simulink model "CusakisME4901arcs2"  (R2013a)
settings: Solver=ode4  StartTime=0.0  StopTime=inf  FixedStep=0.01  RelTol=1e-3
InitFcn:
  | start_EEVSCube2
  | 
  | %links masses
  | 
  | m=20;%Kg
  | 
  | l=1;%meter
  | 
  | w=0.08;
  | 
  | I=(1/12)*m*(l^2); %moment of inertia
  | 
  | %estimation error
  | 
  | mn=20+m*0.05;
  | In=I+I*0.1;
  | 
  | %controls
  | 
  | a=0.7; %singularity positive gain
  | 
  | %Chaser
  | mb=100;%kg
  | lc=2;%meters
  | lb=lc/2;%meter distance 1joint to CM
  | Ib=(1/12)*mb*(lc^2+lc^2);
  | 
  | %Target
  | 
  | mt=750;%kg target mass
  | lt=1;%meter  side lenght
  | It=(1/6)*(lt^2)*mt;
  | 
  | %Target Initial Conitions
  | 
  | x_t=2;
  | y_t=2;
  | theta_t=0.7853;
  | 
  | Init_t=[x_t;y_t;theta_t;0;0;0];
  | Iinv=pinv(eye(3)*It);
StopFcn:
  | figure(1)
  | subplot(2,1,1)
  | hold on
  | plot(time,kinetic,'g')
  | grid on
  | title('Kinetic Energy vs Time')
  | xlabel('Time')
  | ylabel('Kinetic Energy')
  | hold off
  | 
  | subplot(2,1,2)
  | hold on
  | plot(time,power,'g')
  | grid on
  | title('Power Consumption vs Time')
  | xlabel('Time')
  | ylabel('Power')
  | hold off
  | 
  | chasermapping=[-1,1;-1,-1;1,-1;1,1;-1,1];
  | targetmapping=[1.293,2;2,2.707;2.707,2;2,1.293;1.293,2];
  | 
  | figure(3)
  | hold on
  | plot(EEstate(:,1),EEstate(:,2),'g')
  | plot(targetmapping(:,1),targetmapping(:,2),'r')
  | plot(chasermapping(:,1),chasermapping(:,2),'b')
  | grid on
  | title('End Effector Path')
  | xlabel('X Axis (m)')
  | ylabel('Y Axis (m)')
  | hold off
  | 
  | 
  | figure(4)
  | subplot(2,1,1)
  | hold on
  | plot(time,qqd(:,1),'g')
  | plot(time,qqd(:,2),'r')
  | plot(time,qqd(:,3),'b')
  | grid on
  | title('Theta vs Time')
  | xlabel('Time (sec)')
  | ylabel('Theta (rad)')
  | legend( 'Theta1 ' , ' Theta2 ' , ' Theta3')
  | hold off
  | 
  | subplot(2,1,2)
  | hold on
  | plot(time,qqd(:,4),'g')
  | plot(time,qqd(:,5),'r')
  | plot(time,qqd(:,6),'b')
  | grid on
  | legend( 'Omega1 ' , ' Omega2 ', ' Omega3 ' )
  | title('Omega vs Time')
  | xlabel('Time (sec)')
  | ylabel('Omega (rad/s)')
values from neighbouring files (symbols this model uses):
  D = sqrt((Xf(1)-Xi(1))^2+(Xf(2)-Xi(2))^2)    [Arcpaths.m]
undefined symbols (not defined in the file or in its folder): mesh_A, mesh_B, serial
libraries: instrumentlib x5, simulink x3, vrlib x2, dspinverses x1, aerolibanimutils x1
(part 4 of 4)

== matlab function CusakisME4901arcs2/Hardware Interface Comuincation/rad to Arm/MATLAB Function3 ==
  data: u input; y output
function y = fcn(u)
%#codegen
udeg=u*180/pi;

%degrees to arduino angles..(avoids negative numbers)
y = (udeg+180)*10;

== matlab function CusakisME4901arcs2/Hardware Interface Comuincation/rad to Arm/MATLAB Function4 ==
  data: u input; y output
function y = fcn(u)
%#codegen
udeg=u*180/pi;

%degrees to arduino angles..(avoids negative numbers)
y = (udeg+180)*10;

== matlab function CusakisME4901arcs2/Hardware Interface Comuincation/rad to Arm/MATLAB Function5 ==
  data: u input; y output
function y = fcn(u)
%#codegen
udeg=u*180/pi;

%degrees to arduino angles..(avoids negative numbers)
y = (udeg+180)*10;

== matlab function CusakisME4901arcs2/Hardware Interface Comuincation/rad to Arm/MATLAB Function ==
  data: Base input; HiBase output; M1 input; LoBase output; HiM1 output; LoM1 output; M2 input; M3 input; End input; HiM2 output; LoM2 output; HiM3 output; LoM3 output; HiEnd output; LoEnd output; other input; HiO output; LoO output
function [HiBase,LoBase,HiM1,LoM1,HiM2,LoM2,HiM3,LoM3,HiEnd,LoEnd,HiO,LoO] = fcn(Base,M1,M2,M3,End,other)
%#codegen


BaseV=typecast(int16(Base),'uint8');
M1V=typecast(int16(M1),'uint8');
M2V=typecast(int16(M2),'uint8');
M3V=typecast(int16(M3),'uint8');
EndV=typecast(int16(End),'uint8');
OtherV=typecast(int16(other),'uint8');


HiBase=BaseV(2);
LoBase=BaseV(1);
HiM1=M1V(2);
LoM1=M1V(1);
HiM2=M2V(2);
LoM2=M2V(1);
HiM3=M3V(2);
LoM3=M3V(1);
HiEnd=EndV(2);
LoEnd=EndV(1);
HiO=OtherV(2);
LoO=OtherV(1);

== matlab function CusakisME4901arcs2/Hardware Interface Comuincation/rad to Arm/MATLAB Function14 ==
  data: data input; checksum output
function checksum = Checksum(data)
% Calculates checksum of command signal

data = int16(data);
tempsum = sum(data);
temp = 255 - mod(tempsum,256);

checksum = uint8(temp);

== matlab function CusakisME4901arcs2/Hardware Interface Comuincation/rad to Arm/MATLAB Function6 ==
  data: u input; y output
function y = fcn(u)
%#codegen
udeg=u*180/pi;

%degrees to arduino angles..(avoids negative numbers)
y = (udeg+180)*10;

== matlab function CusakisME4901arcs2/Hardware Interface Comuincation/mm//sec to IRobot Comm/MATLAB Function ==
  data: VelR input; HiR output; VelL input; LoR output; HiL output; LoL output
function [HiR,LoR,HiL,LoL] = fcn(VelR,VelL)
%#codegen


%max velocity 500 mm/s 0.5 m/s


R=typecast(int16(VelR),'uint8');
 %typecast(int16(-200),'uint8')
 
HiR=R(2);
LoR=R(1);

L=typecast(int16(VelL),'uint8');
 %typecast(int16(-200),'uint8')
 
HiL=L(2);
LoL=L(1);

== matlab function CusakisME4901arcs2/Hardware Interface Comuincation/Roomba Dynamics/MATLAB Function ==
  data: SCtranslation input; baseoutm input; Velm input; timer input; NewPos input; basem input; Vel output; timem output; NP output; base output; baseout output; enable output
function [Vel,timem,NP,base,baseout,enable] = fcn(SCtranslation,baseoutm,Velm,timer,NewPos,basem)
%#codegen

%This is an approximate model necessary when VICON is not available
%is based on a time estimation for the maneuver (commands until should be
%there)

%Velocity Vector

%Inputs

R=0;
Sl=0;
Sr=0;
r=0.13;
if timer==0
    
    
    Rotation=[cos(basem) -sin(basem); sin(basem) cos(basem)];
    
    Xf=Rotation*[SCtranslation(1);SCtranslation(2)];
    Xi=Rotation*NewPos;    

    D=sqrt((Xf(1)-Xi(1))^2+(Xf(2)-Xi(2))^2);
    if abs(Xf(2)-Xi(2))>0
    alpha=asin((Xf(2)-Xi(2))/D);
    else
    alpha=0;  
    end 
    if Xf(1)>Xi(1) && Xf(2)>Xi(2)
        R=(D/2)*(1/(sin((pi-2*alpha)/2)));       
        Sl=(pi-2*alpha)*(R+r);
        Sr=(pi-2*alpha)*(R-r);
    elseif Xf(1)<Xi(1) && Xf(2)>Xi(2)
        R=(D/2)*(1/(sin((pi-2*alpha)/2)));
        Sl=(pi-2*alpha)*(R-r);
        Sr=(pi-2*alpha)*(R+r);
    elseif Xf(1)<Xi(1) && Xf(2)<Xi(2)
        R=(D/2)*(1/(sin((pi+2*alpha)/2)));
        Sl=-(pi+2*alpha)*(R-r);
        Sr=-(pi+2*alpha)*(R+r);
    elseif  Xf(1)>Xi(1) && Xf(2)<Xi(2)
        R=(D/2)*(1/(sin((pi+2*alpha)/2)));
        Sl=-(pi+2*alpha)*(R+r);
        Sr=-(pi+2*alpha)*(R-r);
    end
    base =(2*alpha)+basem; %in rad
    baseout=baseoutm+basem/200;
    NP=[SCtranslation(1);SCtranslation(2)];
    %Rotation time at 0.5 m/s
    Vel=[(Sr*1000)/2;(Sl*1000)/2];
    timem=timer+0.01;
    enable=1;
elseif timer>=0.01 && timer<=2  
    Vel=Velm;
    NP=NewPos;
    base=basem;
    baseout=baseoutm+basem/200;
    timem=timer+0.01;
    enable=0;
elseif timer>2 && timer<=3  % zero out the difference between base and Roomba
    Sl=-(basem)*(r);
    Sr=(basem)*(r);
    Vel=[(Sr*1000)/1;(Sl*1000)/1];
    NP=NewPos;
    base=basem; %Resets the base attitude
    baseout=baseoutm-(base/100);
    timem=timer+0.01;
    enable=0;    
else %timem=3.01
    Vel=[0;0];
    NP=NewPos;
    base=0;
    baseout=base;
    timem=0;
    enable=0;
end
